simulink model "linmodel"  (R2018a)
settings: Solver=FixedStepAuto  StartTime=0.0  StopTime=5  FixedStep=.001  RelTol=1e-3
values from neighbouring files (symbols this model uses):
  A = eval(subs(A_sym,{x(1),x(2),x(3),x(4), u},{x0(1),x0(2),x0(3),x0(4), u0}))    [linmodgen.m]    (also in matsim.m = [0, 0, 1, 0; nonlinsim.m = eval(subs(A_sym,{x(1),x(2),x(3),x(4)},{x0(1),x0(2),x0(3),x0()
  B = eval(subs(B_sym,{x(1),x(2),x(3),x(4), u},{x0(1),x0(2),x0(3),x0(4), u0}))    [linmodgen.m]    (also in matsim.m = [0; nonlinsim.m = eval(subs(B_sym,{x(1),x(2),x(3),x(4)},{x0(1),x0(2),x0(3),x0()
  C = eval(subs(C_sym,{x(1),x(2),x(3),x(4), u},{x0(1),x0(2),x0(3),x0(4), u0}))    [linmodgen.m]    (also in matsim.m = eye(4); nonlinsim.m = eval(subs(C_sym,{x(1),x(2),x(3),x(4)},{x0(1),x0(2),x0(3),x0()
  D = eval(subs(D_sym,{x(1),x(2),x(3),x(4), u},{x0(1),x0(2),x0(3),x0(4), u0}))    [linmodgen.m]    (also in matsim.m = zeros(4,1); nonlinsim.m = eval(subs(D_sym,{x(1),x(2),x(3),x(4)},{x0(1),x0(2),x0(3),x0()
  init_conditions = [0, deg2rad(10),0,0]    [matsim.m]
  umax = 1 * ulim    (= 3)    [matsim.m]
  umin = -1 * ulim    (= -3)    [matsim.m]
undefined symbols (not defined in the file or in its folder): K
settings Model: Creator=lucas  LastModifiedBy=lucas
settings OptimizationCC: DefaultParameterBehavior=Inlined  UseDivisionForNetSlopeComputation=on  UseFloatMulNetSlope=on  InlineInvariantSignals=on  PassReuseOutputArgsAs=Individual arguments  ZeroExternalMemoryAtStartup=off  ZeroInternalMemoryAtStartup=off  NoFixptDivByZeroProtection=on  EfficientFloat2IntCast=on  LifeSpan=1  OptimizeBlockOrder=speed  DifferentSizesBufferReuse=on
settings DebuggingCC: ParameterTunabilityLossMsg=error
settings HardwareCC: ProdBitPerPointer=32  ProdBitPerSizeT=32  ProdBitPerPtrDiffT=32  ProdLargestAtomicInteger=Long  ProdLargestAtomicFloat=Double  ProdWordSize=32  ProdLongLongMode=on  ProdHWDeviceType=ARM Compatible->ARM Cortex
settings SFSimCC: MATLABDynamicMemAlloc=off
settings RTWCC: SystemTargetFile=ert.tlc  TemplateMakefile=ert_default_tmf  GenerateReport=on  IncludeHyperlinkInReport=on  LaunchReport=on  GenerateTraceInfo=on  GenerateTraceReport=on  GenerateTraceReportSl=on  GenerateTraceReportSf=on  GenerateTraceReportEml=on  GenerateCodeMetricsReport=on
settings CodeAppCC: ForceParamTrailComments=on  IgnoreCustomStorageClasses=off  OperatorAnnotations=on  SimulinkDataObjDesc=on  SFDataObjDesc=on  CustomSymbolStrGlobalVar=rt$N$M  CustomSymbolStrType=$N$M  CustomSymbolStrFcn=$N$M$F  CustomSymbolStrMacro=$N$M  InsertBlockDesc=on
settings ERTTargetCC: TargetLangStandard=C99 (ISO)  GenerateSampleERTMain=on  IncludeMdlTerminateFcn=off  CombineSignalStateStructs=on  SupportAbsoluteTime=off  SupportComplex=off  SupportContinuousTime=on  InlinedParameterPlacement=NonHierarchical  ERTCustomFileTemplate=example_file_process.tlc  ERTFilePackagingFormat=CompactWithDataFile

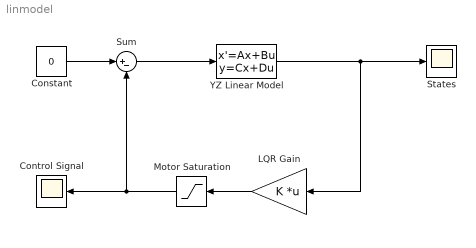
== system linmodel ==
  Constant : Constant  Value=0
  Control Signal : Scope
  LQR Gain : Gain  Gain=K  Multiplication=Matrix(K*u)
  Motor Saturation : Saturate  UpperLimit=umax  LowerLimit=umin
  States : Scope
  Sum : Sum  Inputs=|+-
  YZ Linear Model : StateSpace  A=A  B=B  C=C  D=D  InitialCondition=init_conditions  ContinuousStateAttributes=['phi', 'theta', 'dphi', 'dtheta']
  wires:
  YZ Linear Model/1 -> States/1, LQR Gain/1
  Constant/1 -> Sum/1
  Sum/1 -> YZ Linear Model/1
  LQR Gain/1 -> Motor Saturation/1
  Motor Saturation/1 -> Control Signal/1, Sum/2
